simulink model "validation_simulink"  (R2021a)
settings: Solver=ode4  StartTime=-1.2  StopTime=1.19  RelTol=1e-3
values from neighbouring files (symbols this model uses):
  K = 10^(Kdb/20)    [frequency_response.m]
  tau = 1/(2*pi*(ww(find(squeeze(gww)<=tau_gain, 1, 'first'))))    [frequency_response.m]    (also in ploter_bode.m = get_tau_area)
settings Model: Creator=carol  LastModifiedBy=carol

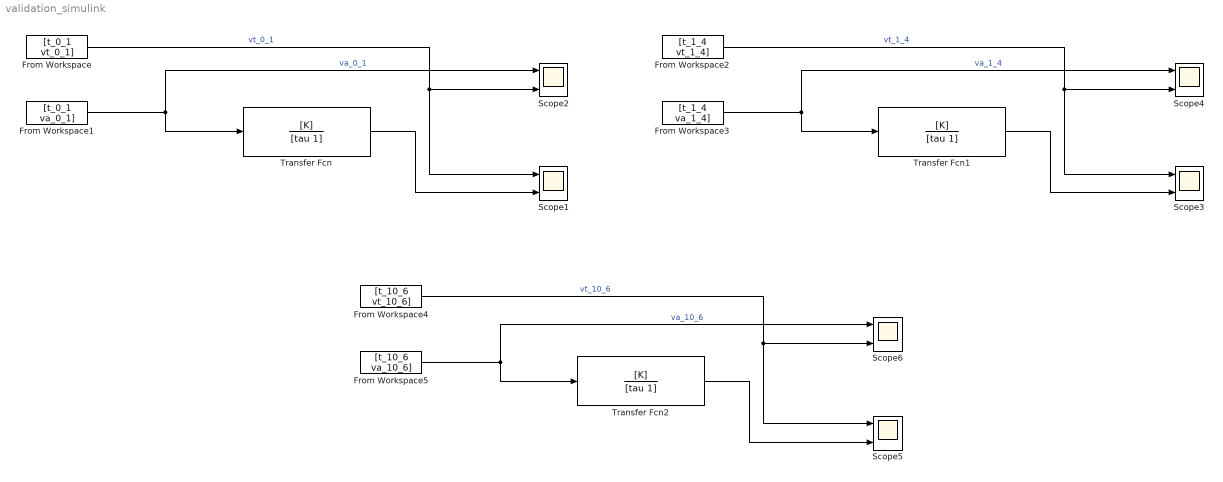
== system validation_simulink ==
  From Workspace : FromWorkspace  VariableName=[t_0_1 vt_0_1]  OutDataTypeStr=double
  From Workspace1 : FromWorkspace  VariableName=[t_0_1 va_0_1]  OutDataTypeStr=double
  From Workspace2 : FromWorkspace  VariableName=[t_1_4 vt_1_4]  OutDataTypeStr=double
  From Workspace3 : FromWorkspace  VariableName=[t_1_4 va_1_4]  OutDataTypeStr=double
  From Workspace4 : FromWorkspace  VariableName=[t_10_6 vt_10_6]  OutDataTypeStr=double
  From Workspace5 : FromWorkspace  VariableName=[t_10_6 va_10_6]  OutDataTypeStr=double
  Scope{1..6} (6 alike) : Scope  NumInputPorts=2
  Transfer Fcn : TransferFcn  Numerator=[K]  Denominator=[tau 1]
  Transfer Fcn1 : TransferFcn  Numerator=[K]  Denominator=[tau 1]
  Transfer Fcn2 : TransferFcn  Numerator=[K]  Denominator=[tau 1]
  wires:
  From Workspace/1 -> Scope1/1, Scope2/2  "vt_0_1"
  Transfer Fcn/1 -> Scope1/2
  From Workspace1/1 -> Transfer Fcn/1, Scope2/1  "va_0_1"
  From Workspace3/1 -> Transfer Fcn1/1, Scope4/1  "va_1_4"
  From Workspace2/1 -> Scope3/1, Scope4/2  "vt_1_4"
  Transfer Fcn1/1 -> Scope3/2
  From Workspace5/1 -> Transfer Fcn2/1, Scope6/1  "va_10_6"
  From Workspace4/1 -> Scope5/1, Scope6/2  "vt_10_6"
  Transfer Fcn2/1 -> Scope5/2
